simulink model "tb_adc_5g_D3"  (Simulink 7.0)
settings: Solver=ode45  StartTime=0.0  StopTime=2000  RelTol=1e-3
libraries: xbsIndex_r4 x125, simulink x36, dspsigops x20, xps_library x2, casper_library x1
(part 1 of 2)
settings Model: Creator=user  LastModifiedBy=homin
settings DebuggingCC: SaveWithParameterizedLinksMsg=none

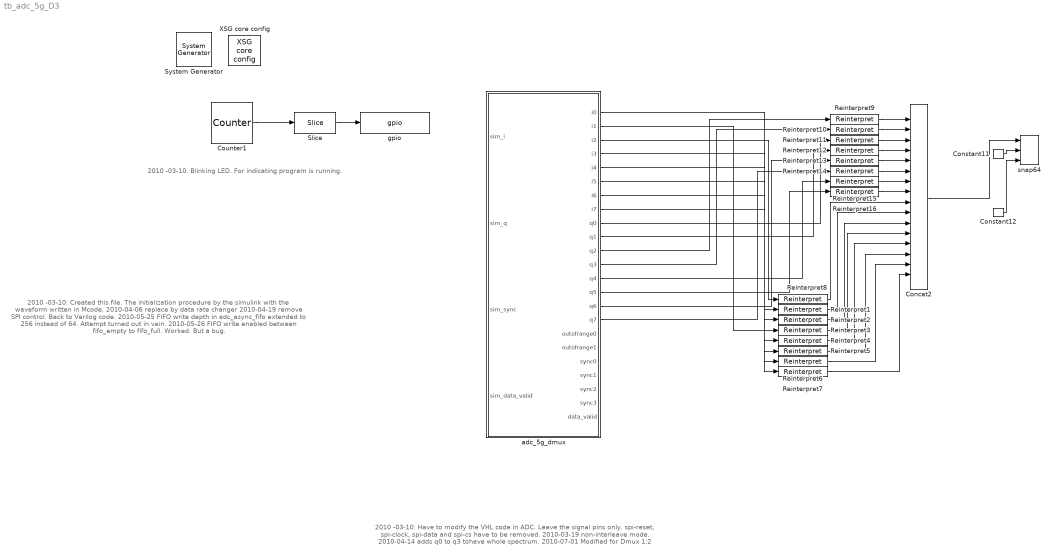
== system tb_adc_5g_D3 ==
  note: 2010 -03-10:
      | Blinking LED. For indicating program is running.
  note: 2010 -03-10:
      | Have to modify the VHL code in ADC. Leave the signal pins only. spi-reset,
      | spi-clock, spi-data and spi-cs have to be removed.
      | 2010-03-19
      | non-interleave mode.
      | 2010-04-14
      | adds q0 to q3 tohave whole spectrum.
      | 2010-07-01
      | Modified for Dmux 1:2
  note: 2010 -03-10:
      | Created this file. The initialization procedure by the simulink with
      | the waveform written in Mcode.
      | 2010-04-06
      | replace by data rate changer
      | 2010-04-19
      | remove SPI control. Back to Verilog code.
      | 2010-05-25
      | FIFO write depth in adc_async_fifo extended to 256 instead of 64. Attempt turned out in vein.
      | 2010-05-26
      | FIFO write enabled between fifo_empty to fifo_full. Worked. But a bug.
  " System Generator" : xbsIndex_r4/ System Generator  Tag=genX  SystemSampleTime=-1  xilinxfamily=virtex5  part=xc5vsx95t  speed=-1  package=ff1136  synthesis_tool=XST  clock_wrapper=Clock Enables  directory=./tb_adc_5g_D3/sysgen  testbench=off  simulink_period=1  sysclk_period=3.3333  dcm_input_clock_period=100  incr_netlist=off  trim_vbits=Everywhere in SubSystem  dbl_ovrd=According to Block Masks  core_generation=According to Block Masks  run_coregen=off  deprecated_control=off  eval_field=0  block_type=sysgen
      settings: block_version=10.1.3
  Concat2 : xbsIndex_r4/Concat  num_inputs=16  dbl_ovrd=off  block_type=concat
      settings: block_version=10.1.3
  Constant11 : xbsIndex_r4/Constant  arith_type=Boolean  const=1  n_bits=16  bin_pt=14  explicit_period=on  period=1  equ=P=C  opselect=C  inp2=PCIN>>17  opr=+  inp1=P  carry=CIN  dbl_ovrd=off  block_type=constant
  Constant12 : xbsIndex_r4/Constant  arith_type=Boolean  const=1  n_bits=16  bin_pt=14  explicit_period=on  period=1  equ=P=C  opselect=C  inp2=PCIN>>17  opr=+  inp1=P  carry=CIN  dbl_ovrd=off  block_type=constant
  Counter1 : xbsIndex_r4/Counter  cnt_type=Free Running  cnt_to=Inf  operation=Up  start_count=0  cnt_by_val=1  arith_type=Unsigned  n_bits=27  bin_pt=0  load_pin=off  rst=off  en=off  explicit_period=on  period=1  dbl_ovrd=off  use_behavioral_HDL=off  use_rpm=off  implementation=Fabric  block_type=counter
  Reinterpret{1..16} (16 alike) : xbsIndex_r4/Reinterpret  force_arith_type=on  arith_type=Unsigned  force_bin_pt=on  bin_pt=0  block_type=reinterpret
      settings: infoedit="Changes signal type without altering the binary representation.   You can changed the signal between signed and unsigned, and relocate the binary point.<P><P>Hardware notes: In hardware this block costs nothing.<P><P>Example:  Suppose the input is 6 bits wide, signed, with 2 fractional bits, and the output is forced to unsigned with 0 fractional bits.  Then an input of -2.0 (1110.00 in binary 2's complement) becomes an output of 56 (111000 in binary)."  block_version=10.1.3
  Slice : xbsIndex_r4/Slice  nbits=1  boolean_output=on  mode=Lower Bit Location + Width  bit1=27  base1=MSB of Input  bit0=26  base0=LSB of Input  dbl_ovrd=off  block_type=slice
      settings: infoedit="Extracts a given range of bits from each input sample and presents it at the output.  The output type is ordinarily unsigned with binary point at zero, but can be Boolean when the slice is one bit wide.<P><P>Hardware notes: In hardware this block costs nothing."  block_version=10.1.3
  XSG core config : xps_library/XSG core config  Tag=xps:xsg  SystemSampleTime=-1  hw_sys=ROACH:sx95t  ibob_linux=off  clk_src=adc0_clk  iBOB_clk_src=sys_clk  BEE2_ctrl_clk_src=sys_clk  BEE2_usr_clk_src=sys_clk  ROACH_clk_src=adc0_clk  CORR_clk_src=sys_clk  gpio_clk_io_group=iBOB:sma  gpio_clk_bit_index=0  clk_rate=300  sample_period=1  synthesis_tool=XST  mpc_type=powerpc440_ext
  adc_5g_dmux : Subsystem  Tag=xps:adc_5g_dmux  mask(adc){adc_brd=adc0, adc_clk_rate=1200, adc_interleave=off, sample_period=1}
      mask prompts: adc_brd "ADC board"; adc_clk_rate "ADC clock rate (MHz)"; adc_interleave "ADC interleave mode"; sample_period "Sample period"
      mask help: The ADC block converts analog inputs to digital outputs. Every clock cycle, the inputs are sampled and digitized to 8 bit binary point numbers in the range of [-1, 1) and are then output by the adc.
      mask init:
      | adc_5g_mask;
      mask Help: eval('xlWeb([getenv(''MLIB_ROOT''), ''\doc\html\sys_adc\sys_adc.html''])')
      mask StyleString: popup(adc0|adc1),edit,checkbox,edit
  gpio : xps_library/gpio  Tag=xps:gpio  SystemSampleTime=-1  io_group=ROACH:led  io_dir=out  arith_type=Boolean  bitwidth=1  bin_pt=0  bit_index=1  sample_period=1  use_single_ended=off  use_ddr=off  reg_iob=on  reg_clk_phase=0  termination=None
      link override convert: arith_type=Boolean  n_bits=1  bin_pt=0
  snap64 : casper_library/Scopes/snap64  SystemSampleTime=-1  nsamples=11
      link override addr/convert: arith_type=Unsigned  n_bits=32  bin_pt=0
      link override bram_lsb/convert_din: arith_type=Unsigned
      link override bram_lsb/mem/sim_data_in: arith_type=Unsigned
      link override bram_lsb/tb_adc_5g_D1_snap64_bram_lsb_data_out: arith_type=Unsigned
      link override bram_lsb/tb_adc_5g_D2_snap64_bram_lsb_data_out: arith_type=Unsigned
      link override bram_lsb/tb_adc_5g_D3_snap64_bram_lsb_data_out: arith_type=Unsigned
      link override bram_lsb/tb_adc_5g_spi_V3_snap64_bram_lsb_data_out: arith_type=Unsigned
      link override bram_lsb/tb_adc_5g_spi_V5_snap64_bram_lsb_data_out: arith_type=Unsigned
      link override bram_lsb/tb_adc_5g_spi_rw2_snap64_bram_lsb_data_out: arith_type=Unsigned
      link override bram_lsb/tut6_snap64_bram_lsb_data_out: arith_type=Unsigned
      link override bram_msb/convert_din: arith_type=Unsigned
      link override bram_msb/mem/sim_data_in: arith_type=Unsigned
      link override bram_msb/tb_adc_5g_D1_snap64_bram_msb_data_out: arith_type=Unsigned
      link override bram_msb/tb_adc_5g_D2_snap64_bram_msb_data_out: arith_type=Unsigned
      link override bram_msb/tb_adc_5g_D3_snap64_bram_msb_data_out: arith_type=Unsigned
      link override bram_msb/tb_adc_5g_spi_V3_snap64_bram_msb_data_out: arith_type=Unsigned
      link override bram_msb/tb_adc_5g_spi_V5_snap64_bram_msb_data_out: arith_type=Unsigned
      link override bram_msb/tb_adc_5g_spi_rw2_snap64_bram_msb_data_out: arith_type=Unsigned
      link override bram_msb/tut6_snap64_bram_msb_data_out: arith_type=Unsigned
      link override ctrl/tb_adc_5g_D1_snap64_ctrl_user_data_out: arith_type=Unsigned  n_bits=32  bin_pt=0  period=1
      link override ctrl/tb_adc_5g_D2_snap64_ctrl_user_data_out: arith_type=Unsigned  n_bits=32  bin_pt=0  period=1
      link override ctrl/tb_adc_5g_D3_snap64_ctrl_user_data_out: arith_type=Unsigned  n_bits=32  bin_pt=0  period=1
      link override ctrl/tb_adc_5g_spi_V3_snap64_ctrl_user_data_out: arith_type=Unsigned  n_bits=32  bin_pt=0  period=1
      link override ctrl/tb_adc_5g_spi_V5_snap64_ctrl_user_data_out: arith_type=Unsigned  n_bits=32  bin_pt=0  period=1
      link override ctrl/tb_adc_5g_spi_rw2_snap64_ctrl_user_data_out: arith_type=Unsigned  n_bits=32  bin_pt=0  period=1
      link override ctrl/tut6_snap64_ctrl_user_data_out: arith_type=Unsigned  n_bits=32  bin_pt=0  period=1
  wires:
  Counter1/1 -> Slice/1
  Slice/1 -> gpio/1
  Reinterpret9/1 -> Concat2/1
  Reinterpret10/1 -> Concat2/2
  Reinterpret11/1 -> Concat2/3
  Reinterpret12/1 -> Concat2/4
  Reinterpret13/1 -> Concat2/5
  Reinterpret14/1 -> Concat2/6
  Reinterpret15/1 -> Concat2/7
  Reinterpret16/1 -> Concat2/8
  Concat2/1 -> snap64/1
  Constant11/1 -> snap64/2
  Constant12/1 -> snap64/3
  Reinterpret8/1 -> Concat2/9
  Reinterpret1/1 -> Concat2/10
  Reinterpret2/1 -> Concat2/11
  Reinterpret3/1 -> Concat2/12
  Reinterpret4/1 -> Concat2/13
  Reinterpret5/1 -> Concat2/14
  Reinterpret6/1 -> Concat2/15
  Reinterpret7/1 -> Concat2/16
  adc_5g_dmux/11(q2) -> Reinterpret9/1
  adc_5g_dmux/12(q3) -> Reinterpret10/1
  adc_5g_dmux/9(q0) -> Reinterpret11/1
  adc_5g_dmux/10(q1) -> Reinterpret12/1
  adc_5g_dmux/13(q4) -> Reinterpret15/1
  adc_5g_dmux/14(q5) -> Reinterpret16/1
  adc_5g_dmux/15(q6) -> Reinterpret13/1
  adc_5g_dmux/16(q7) -> Reinterpret14/1
  adc_5g_dmux/3(i2) -> Reinterpret8/1
  adc_5g_dmux/4(i3) -> Reinterpret1/1
  adc_5g_dmux/1(i0) -> Reinterpret2/1
  adc_5g_dmux/2(i1) -> Reinterpret3/1
  adc_5g_dmux/7(i6) -> Reinterpret4/1
  adc_5g_dmux/8(i7) -> Reinterpret5/1
  adc_5g_dmux/5(i4) -> Reinterpret6/1
  adc_5g_dmux/6(i5) -> Reinterpret7/1

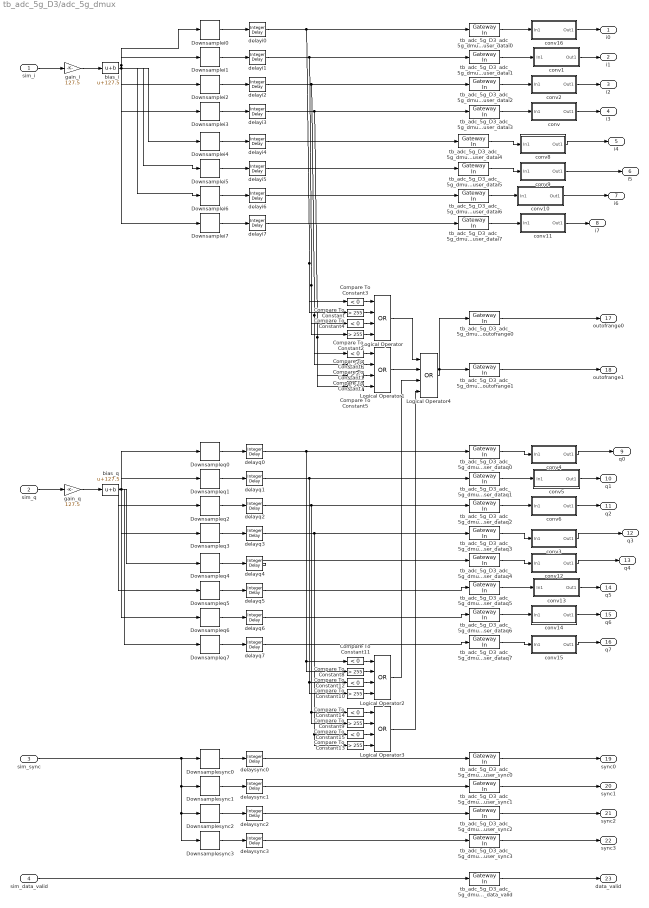
== system tb_adc_5g_D3/adc_5g_dmux ==
  sim_i : Inport  SampleTime=sample_period/4
  sim_q : Inport  Port=2  SampleTime=sample_period/4
  sim_sync : Inport  Port=3  SampleTime=sample_period/4  OutDataType=sfix(16)  OutScaling=2^0
  sim_data_valid : Inport  Port=4  SampleTime=sample_period/4  OutDataType=sfix(16)  OutScaling=2^0
  Compare To Constant{,1..2,5,8..10,13} (8 alike) : simulink/Logic and Bit Operations/Compare To Constant  SystemSampleTime=-1  relop=>  const=255  LogicOutDataTypeMode=boolean  ZeroCross=off
  Compare To Constant{3..4,6..7,11..12,14..15} (8 alike) : simulink/Logic and Bit Operations/Compare To Constant  SystemSampleTime=-1  relop=<  const=0  LogicOutDataTypeMode=boolean  ZeroCross=off
  Downsamplei0 : dspsigops/Downsample  N=4  phase=0  ic=0  smode=Allow multirate  fmode=Maintain input frame size
  Downsamplei1 : dspsigops/Downsample  N=4  phase=1  ic=0  smode=Allow multirate  fmode=Maintain input frame size
  Downsamplei2 : dspsigops/Downsample  N=4  phase=2  ic=0  smode=Allow multirate  fmode=Maintain input frame size
  Downsamplei3 : dspsigops/Downsample  N=4  phase=3  ic=0  smode=Allow multirate  fmode=Maintain input frame size
  Downsamplei4 : dspsigops/Downsample  N=4  phase=0  ic=0  smode=Allow multirate  fmode=Maintain input frame size
  Downsamplei5 : dspsigops/Downsample  N=4  phase=1  ic=0  smode=Allow multirate  fmode=Maintain input frame size
  Downsamplei6 : dspsigops/Downsample  N=4  phase=2  ic=0  smode=Allow multirate  fmode=Maintain input frame size
  Downsamplei7 : dspsigops/Downsample  N=4  phase=3  ic=0  smode=Allow multirate  fmode=Maintain input frame size
  Downsampleq0 : dspsigops/Downsample  N=4  phase=0  ic=0  smode=Allow multirate  fmode=Maintain input frame size
  Downsampleq1 : dspsigops/Downsample  N=4  phase=1  ic=0  smode=Allow multirate  fmode=Maintain input frame size
  Downsampleq2 : dspsigops/Downsample  N=4  phase=2  ic=0  smode=Allow multirate  fmode=Maintain input frame size
  Downsampleq3 : dspsigops/Downsample  N=4  phase=3  ic=0  smode=Allow multirate  fmode=Maintain input frame size
  Downsampleq4 : dspsigops/Downsample  N=4  phase=0  ic=0  smode=Allow multirate  fmode=Maintain input frame size
  Downsampleq5 : dspsigops/Downsample  N=4  phase=1  ic=0  smode=Allow multirate  fmode=Maintain input frame size
  Downsampleq6 : dspsigops/Downsample  N=4  phase=2  ic=0  smode=Allow multirate  fmode=Maintain input frame size
  Downsampleq7 : dspsigops/Downsample  N=4  phase=3  ic=0  smode=Allow multirate  fmode=Maintain input frame size
  Downsamplesync0 : dspsigops/Downsample  N=4  phase=0  ic=0  smode=Allow multirate  fmode=Maintain input frame size
  Downsamplesync1 : dspsigops/Downsample  N=4  phase=1  ic=0  smode=Allow multirate  fmode=Maintain input frame size
  Downsamplesync2 : dspsigops/Downsample  N=4  phase=2  ic=0  smode=Allow multirate  fmode=Maintain input frame size
  Downsamplesync3 : dspsigops/Downsample  N=4  phase=3  ic=0  smode=Allow multirate  fmode=Maintain input frame size
  Logical Operator{,1..4} (5 alike) : Logic  Operator=OR  Inputs=4  AllPortsSameDT=off  OutDataTypeMode=boolean
  bias_i : Bias  Bias=127.5  SaturateOnIntegerOverflow=on
  bias_q : Bias  Bias=127.5  SaturateOnIntegerOverflow=on
  conv : Subsystem
  conv1 : Subsystem
  conv10 : Subsystem
  conv11 : Subsystem
  conv12 : Subsystem
  conv13 : Subsystem
  conv14 : Subsystem
  conv15 : Subsystem
  conv16 : Subsystem
  conv2 : Subsystem
  conv3 : Subsystem
  conv4 : Subsystem
  conv5 : Subsystem
  conv6 : Subsystem
  conv8 : Subsystem
  conv9 : Subsystem
  delayi0 : simulink/Discrete/Integer Delay  vinit=0.0  samptime=-1  NumDelays=2
  delayi{1..3,5..7} (6 alike) : simulink/Discrete/Integer Delay  vinit=0.0  samptime=-1  NumDelays=1
  delayi4 : simulink/Discrete/Integer Delay  vinit=0.0  samptime=-1  NumDelays=2
  delayq0 : simulink/Discrete/Integer Delay  vinit=0.0  samptime=-1  NumDelays=2
  delayq{1..3,5..7} (6 alike) : simulink/Discrete/Integer Delay  vinit=0.0  samptime=-1  NumDelays=1
  delayq4 : simulink/Discrete/Integer Delay  vinit=0.0  samptime=-1  NumDelays=2
  delaysync0 : simulink/Discrete/Integer Delay  vinit=0.0  samptime=-1  NumDelays=2
  delaysync1 : simulink/Discrete/Integer Delay  vinit=0.0  samptime=-1  NumDelays=1
  delaysync2 : simulink/Discrete/Integer Delay  vinit=0.0  samptime=-1  NumDelays=1
  delaysync3 : simulink/Discrete/Integer Delay  vinit=0.0  samptime=-1  NumDelays=1
  gain_i : Gain  Gain=127.5  SaturateOnIntegerOverflow=on
  gain_q : Gain  Gain=127.5  SaturateOnIntegerOverflow=on
  tb_adc_5g_D3_adc_5g_dmux_user_data_valid : xbsIndex_r4/Gateway In  arith_type=Boolean  n_bits=8  bin_pt=0  quantization="Round  (unbiased: +/- Inf)"  overflow=Saturate  period=sample_period  dbl_ovrd=off  timing_constraint=None  locs_specified=off  LOCs={}  block_type=gatewayin
      settings: infoedit="Gateway in block.  Converts inputs of type Simulink integer, double and fixed point to  Xilinx fixed point type.<P><P>Hardware notes:  In hardware these blocks become top level input ports."  xl_area=[0 0 0 0 8 0 0]  block_version=8.2.02
  tb_adc_5g_D3_adc_5g_dmux_user_datai{0..7} (8 alike) : xbsIndex_r4/Gateway In  arith_type=Unsigned  n_bits=4  bin_pt=0  quantization="Round  (unbiased: +/- Inf)"  overflow=Saturate  period=sample_period  dbl_ovrd=off  timing_constraint=None  locs_specified=off  LOCs={}  block_type=gatewayin
      settings: infoedit="Gateway in block.  Converts inputs of type Simulink integer, double and fixed point to  Xilinx fixed point type.<P><P>Hardware notes:  In hardware these blocks become top level input ports."  xl_area=[0 0 0 0 8 0 0]  block_version=8.2.02
  tb_adc_5g_D3_adc_5g_dmux_user_dataq{0..7} (8 alike) : xbsIndex_r4/Gateway In  arith_type=Unsigned  n_bits=4  bin_pt=0  quantization="Round  (unbiased: +/- Inf)"  overflow=Saturate  period=sample_period  dbl_ovrd=off  timing_constraint=None  locs_specified=off  LOCs={}  block_type=gatewayin
      settings: infoedit="Gateway in block.  Converts inputs of type Simulink integer, double and fixed point to  Xilinx fixed point type.<P><P>Hardware notes:  In hardware these blocks become top level input ports."  xl_area=[0 0 0 0 8 0 0]  block_version=8.2.02
  tb_adc_5g_D3_adc_5g_dmux_user_outofrange0 : xbsIndex_r4/Gateway In  arith_type=Boolean  n_bits=8  bin_pt=0  quantization="Round  (unbiased: +/- Inf)"  overflow=Saturate  period=sample_period  dbl_ovrd=off  timing_constraint=None  locs_specified=off  LOCs={}  block_type=gatewayin
      settings: infoedit="Gateway in block.  Converts inputs of type Simulink integer, double and fixed point to  Xilinx fixed point type.<P><P>Hardware notes:  In hardware these blocks become top level input ports."  xl_area=[0 0 0 0 8 0 0]  block_version=8.2.02
  tb_adc_5g_D3_adc_5g_dmux_user_outofrange1 : xbsIndex_r4/Gateway In  arith_type=Boolean  n_bits=8  bin_pt=0  quantization="Round  (unbiased: +/- Inf)"  overflow=Saturate  period=sample_period  dbl_ovrd=off  timing_constraint=None  locs_specified=off  LOCs={}  block_type=gatewayin
      settings: infoedit="Gateway in block.  Converts inputs of type Simulink integer, double and fixed point to  Xilinx fixed point type.<P><P>Hardware notes:  In hardware these blocks become top level input ports."  xl_area=[0 0 0 0 8 0 0]  block_version=8.2.02
  tb_adc_5g_D3_adc_5g_dmux_user_sync{0..3} (4 alike) : xbsIndex_r4/Gateway In  arith_type=Boolean  n_bits=8  bin_pt=0  quantization="Round  (unbiased: +/- Inf)"  overflow=Saturate  period=sample_period  dbl_ovrd=off  timing_constraint=None  locs_specified=off  LOCs={}  block_type=gatewayin
      settings: infoedit="Gateway in block.  Converts inputs of type Simulink integer, double and fixed point to  Xilinx fixed point type.<P><P>Hardware notes:  In hardware these blocks become top level input ports."  xl_area=[0 0 0 0 8 0 0]  block_version=8.2.02
  i0 : Outport  OutDataType=sfix(16)  OutScaling=2^0
  i1 : Outport  Port=2  OutDataType=sfix(16)  OutScaling=2^0
  i2 : Outport  Port=3  OutDataType=sfix(16)  OutScaling=2^0
  i3 : Outport  Port=4  OutDataType=sfix(16)  OutScaling=2^0
  i4 : Outport  Port=5  OutDataType=sfix(16)  OutScaling=2^0
  i5 : Outport  Port=6  OutDataType=sfix(16)  OutScaling=2^0
  i6 : Outport  Port=7  OutDataType=sfix(16)  OutScaling=2^0
  i7 : Outport  Port=8  OutDataType=sfix(16)  OutScaling=2^0
  q0 : Outport  Port=9  OutDataType=sfix(16)  OutScaling=2^0
  q1 : Outport  Port=10  OutDataType=sfix(16)  OutScaling=2^0
  q2 : Outport  Port=11  OutDataType=sfix(16)  OutScaling=2^0
  q3 : Outport  Port=12  OutDataType=sfix(16)  OutScaling=2^0
  q4 : Outport  Port=13  OutDataType=sfix(16)  OutScaling=2^0
  q5 : Outport  Port=14  OutDataType=sfix(16)  OutScaling=2^0
  q6 : Outport  Port=15  OutDataType=sfix(16)  OutScaling=2^0
  q7 : Outport  Port=16  OutDataType=sfix(16)  OutScaling=2^0
  outofrange0 : Outport  Port=17  OutDataType=sfix(16)  OutScaling=2^0
  outofrange1 : Outport  Port=18  OutDataType=sfix(16)  OutScaling=2^0
  sync0 : Outport  Port=19  OutDataType=sfix(16)  OutScaling=2^0
  sync1 : Outport  Port=20  OutDataType=sfix(16)  OutScaling=2^0
  sync2 : Outport  Port=21  OutDataType=sfix(16)  OutScaling=2^0
  sync3 : Outport  Port=22  OutDataType=sfix(16)  OutScaling=2^0
  data_valid : Outport  Port=23  OutDataType=sfix(16)  OutScaling=2^0
  wires:
  tb_adc_5g_D3_adc_5g_dmux_user_datai0/1 -> conv16/1(In1)
  sim_data_valid/1 -> tb_adc_5g_D3_adc_5g_dmux_user_data_valid/1
  tb_adc_5g_D3_adc_5g_dmux_user_data_valid/1 -> data_valid/1
  tb_adc_5g_D3_adc_5g_dmux_user_sync3/1 -> sync3/1
  tb_adc_5g_D3_adc_5g_dmux_user_sync2/1 -> sync2/1
  delaysync3/1 -> tb_adc_5g_D3_adc_5g_dmux_user_sync3/1
  delaysync2/1 -> tb_adc_5g_D3_adc_5g_dmux_user_sync2/1
  Downsamplesync3/1 -> delaysync3/1
  Downsamplesync2/1 -> delaysync2/1
  tb_adc_5g_D3_adc_5g_dmux_user_sync1/1 -> sync1/1
  delaysync0/1 -> tb_adc_5g_D3_adc_5g_dmux_user_sync0/1
  Downsamplesync1/1 -> delaysync1/1
  Downsamplesync0/1 -> delaysync0/1
  sim_sync/1 -> Downsamplesync3/1, Downsamplesync2/1, Downsamplesync1/1, Downsamplesync0/1
  Compare To Constant5/1 -> Logical Operator1/4
  Compare To Constant7/1 -> Logical Operator1/3
  Compare To Constant1/1 -> Logical Operator1/2
  Compare To Constant6/1 -> Logical Operator1/1
  Compare To Constant2/1 -> Logical Operator/4
  Compare To Constant4/1 -> Logical Operator/3
  Compare To Constant/1 -> Logical Operator/2
  Compare To Constant3/1 -> Logical Operator/1
  tb_adc_5g_D3_adc_5g_dmux_user_outofrange1/1 -> outofrange1/1
  delayq0/1 -> tb_adc_5g_D3_adc_5g_dmux_user_dataq0/1, Compare To Constant8/1, Compare To Constant11/1
  Downsampleq0/1 -> delayq0/1
  delayi0/1 -> Compare To Constant3/1, Compare To Constant/1, tb_adc_5g_D3_adc_5g_dmux_user_datai0/1
  Downsamplei1/1 -> delayi1/1
  Downsamplei2/1 -> delayi2/1
  Downsamplei3/1 -> delayi3/1
  Downsampleq1/1 -> delayq1/1
  Downsampleq2/1 -> delayq2/1
  Downsampleq3/1 -> delayq3/1
  tb_adc_5g_D3_adc_5g_dmux_user_datai1/1 -> conv1/1(In1)
  tb_adc_5g_D3_adc_5g_dmux_user_datai2/1 -> conv2/1(In1)
  tb_adc_5g_D3_adc_5g_dmux_user_datai3/1 -> conv/1(In1)
  tb_adc_5g_D3_adc_5g_dmux_user_outofrange0/1 -> outofrange0/1
  tb_adc_5g_D3_adc_5g_dmux_user_sync0/1 -> sync0/1
  conv16/1(Out1) -> i0/1
  conv1/1(Out1) -> i1/1
  conv2/1(Out1) -> i2/1
  conv/1(Out1) -> i3/1
  tb_adc_5g_D3_adc_5g_dmux_user_dataq0/1 -> conv4/1(In1)
  conv4/1(Out1) -> q0/1
  tb_adc_5g_D3_adc_5g_dmux_user_dataq1/1 -> conv5/1(In1)
  conv5/1(Out1) -> q1/1
  tb_adc_5g_D3_adc_5g_dmux_user_dataq2/1 -> conv6/1(In1)
  conv6/1(Out1) -> q2/1
  tb_adc_5g_D3_adc_5g_dmux_user_dataq3/1 -> conv3/1(In1)
  conv3/1(Out1) -> q3/1
  Downsamplei0/1 -> delayi0/1
  delayi1/1 -> Compare To Constant4/1, Compare To Constant2/1, tb_adc_5g_D3_adc_5g_dmux_user_datai1/1
  delayi2/1 -> Compare To Constant1/1, Compare To Constant6/1, tb_adc_5g_D3_adc_5g_dmux_user_datai2/1
  delayi3/1 -> Compare To Constant5/1, Compare To Constant7/1, tb_adc_5g_D3_adc_5g_dmux_user_datai3/1
  delayq1/1 -> Compare To Constant10/1, Compare To Constant12/1, tb_adc_5g_D3_adc_5g_dmux_user_dataq1/1
  delayq2/1 -> Compare To Constant9/1, Compare To Constant14/1, tb_adc_5g_D3_adc_5g_dmux_user_dataq2/1
  delayq3/1 -> Compare To Constant13/1, Compare To Constant15/1, tb_adc_5g_D3_adc_5g_dmux_user_dataq3/1
  delaysync1/1 -> tb_adc_5g_D3_adc_5g_dmux_user_sync1/1
  Compare To Constant11/1 -> Logical Operator2/1
  Compare To Constant13/1 -> Logical Operator3/4
  Compare To Constant15/1 -> Logical Operator3/3
  Compare To Constant9/1 -> Logical Operator3/2
  Compare To Constant14/1 -> Logical Operator3/1
  Compare To Constant10/1 -> Logical Operator2/4
  Compare To Constant12/1 -> Logical Operator2/3
  Compare To Constant8/1 -> Logical Operator2/2
  Logical Operator4/1 -> tb_adc_5g_D3_adc_5g_dmux_user_outofrange0/1, tb_adc_5g_D3_adc_5g_dmux_user_outofrange1/1
  Logical Operator/1 -> Logical Operator4/1
  Logical Operator1/1 -> Logical Operator4/2
  Logical Operator2/1 -> Logical Operator4/3
  Logical Operator3/1 -> Logical Operator4/4
  sim_i/1 -> gain_i/1
  gain_i/1 -> bias_i/1
  bias_i/1 -> Downsamplei1/1, Downsamplei2/1, Downsamplei3/1, Downsamplei4/1, Downsamplei5/1, Downsamplei6/1, Downsamplei0/1, Downsamplei7/1
  sim_q/1 -> gain_q/1
  gain_q/1 -> bias_q/1
  bias_q/1 -> Downsampleq0/1, Downsampleq1/1, Downsampleq3/1, Downsampleq4/1, Downsampleq2/1, Downsampleq5/1, Downsampleq6/1, Downsampleq7/1
  tb_adc_5g_D3_adc_5g_dmux_user_datai4/1 -> conv8/1(In1)
  delayi4/1 -> tb_adc_5g_D3_adc_5g_dmux_user_datai4/1
  tb_adc_5g_D3_adc_5g_dmux_user_datai5/1 -> conv9/1(In1)
  tb_adc_5g_D3_adc_5g_dmux_user_datai6/1 -> conv10/1(In1)
  tb_adc_5g_D3_adc_5g_dmux_user_datai7/1 -> conv11/1(In1)
  conv8/1(Out1) -> i4/1
  conv9/1(Out1) -> i5/1
  conv10/1(Out1) -> i6/1
  conv11/1(Out1) -> i7/1
  delayi5/1 -> tb_adc_5g_D3_adc_5g_dmux_user_datai5/1
  delayi6/1 -> tb_adc_5g_D3_adc_5g_dmux_user_datai6/1
  delayi7/1 -> tb_adc_5g_D3_adc_5g_dmux_user_datai7/1
  Downsamplei5/1 -> delayi5/1
  Downsamplei6/1 -> delayi6/1
  Downsamplei7/1 -> delayi7/1
  Downsamplei4/1 -> delayi4/1
  tb_adc_5g_D3_adc_5g_dmux_user_dataq4/1 -> conv12/1(In1)
  conv12/1(Out1) -> q4/1
  tb_adc_5g_D3_adc_5g_dmux_user_dataq5/1 -> conv13/1(In1)
  conv13/1(Out1) -> q5/1
  tb_adc_5g_D3_adc_5g_dmux_user_dataq6/1 -> conv14/1(In1)
  conv14/1(Out1) -> q6/1
  tb_adc_5g_D3_adc_5g_dmux_user_dataq7/1 -> conv15/1(In1)
  conv15/1(Out1) -> q7/1
  Downsampleq4/1 -> delayq4/1
  Downsampleq5/1 -> delayq5/1
  Downsampleq6/1 -> delayq6/1
  Downsampleq7/1 -> delayq7/1
  delayq4/1 -> tb_adc_5g_D3_adc_5g_dmux_user_dataq4/1
  delayq5/1 -> tb_adc_5g_D3_adc_5g_dmux_user_dataq5/1
  delayq6/1 -> tb_adc_5g_D3_adc_5g_dmux_user_dataq6/1
  delayq7/1 -> tb_adc_5g_D3_adc_5g_dmux_user_dataq7/1

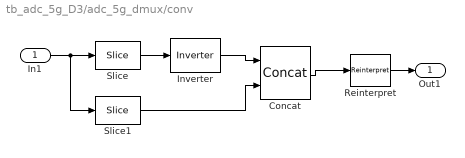
== system tb_adc_5g_D3/adc_5g_dmux/conv ==
  In1 : Inport  OutDataType=sfix(16)  OutScaling=2^0
  Concat : xbsIndex_r4/Concat  num_inputs=2  dbl_ovrd=off  block_type=concat
      settings: block_version=8.2.02
  Inverter : xbsIndex_r4/Inverter  en=off  latency=0  dbl_ovrd=off  block_type=inv
      settings: xl_area=[0, 0, 0, 0, 0, 0, 0]  block_version=8.2.02
  Reinterpret : xbsIndex_r4/Reinterpret  force_arith_type=on  arith_type="Signed  (2's comp)"  force_bin_pt=on  bin_pt=3  block_type=reinterpret
      settings: infoedit="Changes signal type without altering the binary representation.   You can changed the signal between signed and unsigned, and relocate the binary point.<P><P>Hardware notes: In hardware this block costs nothing.<P><P>Example:  Suppose the input is 6 bits wide, signed, with 2 fractional bits, and the output is forced to unsigned with 0 fractional bits.  Then an input of -2.0 (1110.00 in binary 2's complement) becomes an output of 56 (111000 in binary)."  block_version=8.2.02
  Slice : xbsIndex_r4/Slice  nbits=1  boolean_output=off  mode=Upper Bit Location + Width  bit1=0  base1=MSB of Input  bit0=0  base0=LSB of Input  dbl_ovrd=off  block_type=slice
      settings: infoedit="Extracts a given range of bits from each input sample and presents it at the output.  The output type is ordinarily unsigned with binary point at zero, but can be Boolean when the slice is one bit wide.<P><P>Hardware notes: In hardware this block costs nothing."  block_version=8.2.02
  Slice1 : xbsIndex_r4/Slice  nbits=3  boolean_output=off  mode=Lower Bit Location + Width  bit1=0  base1=MSB of Input  bit0=0  base0=LSB of Input  dbl_ovrd=off  block_type=slice
      settings: infoedit="Extracts a given range of bits from each input sample and presents it at the output.  The output type is ordinarily unsigned with binary point at zero, but can be Boolean when the slice is one bit wide.<P><P>Hardware notes: In hardware this block costs nothing."  block_version=8.2.02
  Out1 : Outport  OutDataType=sfix(16)  OutScaling=2^0
  wires:
  In1/1 -> Slice1/1, Slice/1
  Slice/1 -> Inverter/1
  Inverter/1 -> Concat/1
  Slice1/1 -> Concat/2
  Concat/1 -> Reinterpret/1
  Reinterpret/1 -> Out1/1

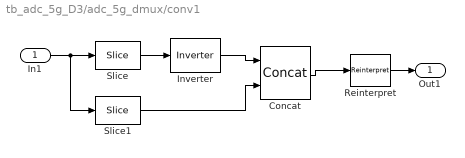
== system tb_adc_5g_D3/adc_5g_dmux/conv1 ==
  In1 : Inport  OutDataType=sfix(16)  OutScaling=2^0
  Concat : xbsIndex_r4/Concat  num_inputs=2  dbl_ovrd=off  block_type=concat
      settings: block_version=8.2.02
  Inverter : xbsIndex_r4/Inverter  en=off  latency=0  dbl_ovrd=off  block_type=inv
      settings: xl_area=[0, 0, 0, 0, 0, 0, 0]  block_version=8.2.02
  Reinterpret : xbsIndex_r4/Reinterpret  force_arith_type=on  arith_type="Signed  (2's comp)"  force_bin_pt=on  bin_pt=3  block_type=reinterpret
      settings: infoedit="Changes signal type without altering the binary representation.   You can changed the signal between signed and unsigned, and relocate the binary point.<P><P>Hardware notes: In hardware this block costs nothing.<P><P>Example:  Suppose the input is 6 bits wide, signed, with 2 fractional bits, and the output is forced to unsigned with 0 fractional bits.  Then an input of -2.0 (1110.00 in binary 2's complement) becomes an output of 56 (111000 in binary)."  block_version=8.2.02
  Slice : xbsIndex_r4/Slice  nbits=1  boolean_output=off  mode=Upper Bit Location + Width  bit1=0  base1=MSB of Input  bit0=0  base0=LSB of Input  dbl_ovrd=off  block_type=slice
      settings: infoedit="Extracts a given range of bits from each input sample and presents it at the output.  The output type is ordinarily unsigned with binary point at zero, but can be Boolean when the slice is one bit wide.<P><P>Hardware notes: In hardware this block costs nothing."  block_version=8.2.02
  Slice1 : xbsIndex_r4/Slice  nbits=3  boolean_output=off  mode=Lower Bit Location + Width  bit1=0  base1=MSB of Input  bit0=0  base0=LSB of Input  dbl_ovrd=off  block_type=slice
      settings: infoedit="Extracts a given range of bits from each input sample and presents it at the output.  The output type is ordinarily unsigned with binary point at zero, but can be Boolean when the slice is one bit wide.<P><P>Hardware notes: In hardware this block costs nothing."  block_version=8.2.02
  Out1 : Outport  OutDataType=sfix(16)  OutScaling=2^0
  wires:
  In1/1 -> Slice1/1, Slice/1
  Slice/1 -> Inverter/1
  Inverter/1 -> Concat/1
  Slice1/1 -> Concat/2
  Concat/1 -> Reinterpret/1
  Reinterpret/1 -> Out1/1

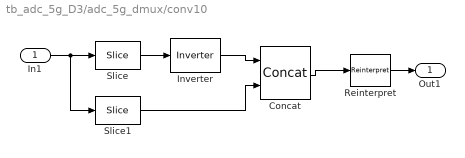
== system tb_adc_5g_D3/adc_5g_dmux/conv10 ==
  In1 : Inport  OutDataType=sfix(16)  OutScaling=2^0
  Concat : xbsIndex_r4/Concat  num_inputs=2  dbl_ovrd=off  block_type=concat
      settings: block_version=8.2.02
  Inverter : xbsIndex_r4/Inverter  en=off  latency=0  dbl_ovrd=off  block_type=inv
      settings: xl_area=[0, 0, 0, 0, 0, 0, 0]  block_version=8.2.02
  Reinterpret : xbsIndex_r4/Reinterpret  force_arith_type=on  arith_type="Signed  (2's comp)"  force_bin_pt=on  bin_pt=3  block_type=reinterpret
      settings: infoedit="Changes signal type without altering the binary representation.   You can changed the signal between signed and unsigned, and relocate the binary point.<P><P>Hardware notes: In hardware this block costs nothing.<P><P>Example:  Suppose the input is 6 bits wide, signed, with 2 fractional bits, and the output is forced to unsigned with 0 fractional bits.  Then an input of -2.0 (1110.00 in binary 2's complement) becomes an output of 56 (111000 in binary)."  block_version=8.2.02
  Slice : xbsIndex_r4/Slice  nbits=1  boolean_output=off  mode=Upper Bit Location + Width  bit1=0  base1=MSB of Input  bit0=0  base0=LSB of Input  dbl_ovrd=off  block_type=slice
      settings: infoedit="Extracts a given range of bits from each input sample and presents it at the output.  The output type is ordinarily unsigned with binary point at zero, but can be Boolean when the slice is one bit wide.<P><P>Hardware notes: In hardware this block costs nothing."  block_version=8.2.02
  Slice1 : xbsIndex_r4/Slice  nbits=3  boolean_output=off  mode=Lower Bit Location + Width  bit1=0  base1=MSB of Input  bit0=0  base0=LSB of Input  dbl_ovrd=off  block_type=slice
      settings: infoedit="Extracts a given range of bits from each input sample and presents it at the output.  The output type is ordinarily unsigned with binary point at zero, but can be Boolean when the slice is one bit wide.<P><P>Hardware notes: In hardware this block costs nothing."  block_version=8.2.02
  Out1 : Outport  OutDataType=sfix(16)  OutScaling=2^0
  wires:
  In1/1 -> Slice1/1, Slice/1
  Slice/1 -> Inverter/1
  Inverter/1 -> Concat/1
  Slice1/1 -> Concat/2
  Concat/1 -> Reinterpret/1
  Reinterpret/1 -> Out1/1

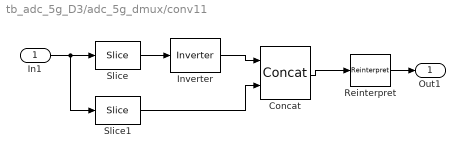
== system tb_adc_5g_D3/adc_5g_dmux/conv11 ==
  In1 : Inport  OutDataType=sfix(16)  OutScaling=2^0
  Concat : xbsIndex_r4/Concat  num_inputs=2  dbl_ovrd=off  block_type=concat
      settings: block_version=8.2.02
  Inverter : xbsIndex_r4/Inverter  en=off  latency=0  dbl_ovrd=off  block_type=inv
      settings: xl_area=[0, 0, 0, 0, 0, 0, 0]  block_version=8.2.02
  Reinterpret : xbsIndex_r4/Reinterpret  force_arith_type=on  arith_type="Signed  (2's comp)"  force_bin_pt=on  bin_pt=3  block_type=reinterpret
      settings: infoedit="Changes signal type without altering the binary representation.   You can changed the signal between signed and unsigned, and relocate the binary point.<P><P>Hardware notes: In hardware this block costs nothing.<P><P>Example:  Suppose the input is 6 bits wide, signed, with 2 fractional bits, and the output is forced to unsigned with 0 fractional bits.  Then an input of -2.0 (1110.00 in binary 2's complement) becomes an output of 56 (111000 in binary)."  block_version=8.2.02
  Slice : xbsIndex_r4/Slice  nbits=1  boolean_output=off  mode=Upper Bit Location + Width  bit1=0  base1=MSB of Input  bit0=0  base0=LSB of Input  dbl_ovrd=off  block_type=slice
      settings: infoedit="Extracts a given range of bits from each input sample and presents it at the output.  The output type is ordinarily unsigned with binary point at zero, but can be Boolean when the slice is one bit wide.<P><P>Hardware notes: In hardware this block costs nothing."  block_version=8.2.02
  Slice1 : xbsIndex_r4/Slice  nbits=3  boolean_output=off  mode=Lower Bit Location + Width  bit1=0  base1=MSB of Input  bit0=0  base0=LSB of Input  dbl_ovrd=off  block_type=slice
      settings: infoedit="Extracts a given range of bits from each input sample and presents it at the output.  The output type is ordinarily unsigned with binary point at zero, but can be Boolean when the slice is one bit wide.<P><P>Hardware notes: In hardware this block costs nothing."  block_version=8.2.02
  Out1 : Outport  OutDataType=sfix(16)  OutScaling=2^0
  wires:
  In1/1 -> Slice1/1, Slice/1
  Slice/1 -> Inverter/1
  Inverter/1 -> Concat/1
  Slice1/1 -> Concat/2
  Concat/1 -> Reinterpret/1
  Reinterpret/1 -> Out1/1

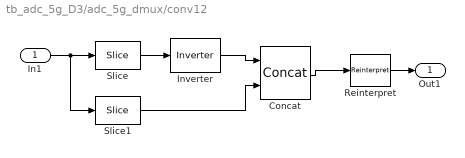
== system tb_adc_5g_D3/adc_5g_dmux/conv12 ==
  In1 : Inport  OutDataType=sfix(16)  OutScaling=2^0
  Concat : xbsIndex_r4/Concat  num_inputs=2  dbl_ovrd=off  block_type=concat
      settings: block_version=8.2.02
  Inverter : xbsIndex_r4/Inverter  en=off  latency=0  dbl_ovrd=off  block_type=inv
      settings: xl_area=[0, 0, 0, 0, 0, 0, 0]  block_version=8.2.02
  Reinterpret : xbsIndex_r4/Reinterpret  force_arith_type=on  arith_type="Signed  (2's comp)"  force_bin_pt=on  bin_pt=3  block_type=reinterpret
      settings: infoedit="Changes signal type without altering the binary representation.   You can changed the signal between signed and unsigned, and relocate the binary point.<P><P>Hardware notes: In hardware this block costs nothing.<P><P>Example:  Suppose the input is 6 bits wide, signed, with 2 fractional bits, and the output is forced to unsigned with 0 fractional bits.  Then an input of -2.0 (1110.00 in binary 2's complement) becomes an output of 56 (111000 in binary)."  block_version=8.2.02
  Slice : xbsIndex_r4/Slice  nbits=1  boolean_output=off  mode=Upper Bit Location + Width  bit1=0  base1=MSB of Input  bit0=0  base0=LSB of Input  dbl_ovrd=off  block_type=slice
      settings: infoedit="Extracts a given range of bits from each input sample and presents it at the output.  The output type is ordinarily unsigned with binary point at zero, but can be Boolean when the slice is one bit wide.<P><P>Hardware notes: In hardware this block costs nothing."  block_version=8.2.02
  Slice1 : xbsIndex_r4/Slice  nbits=3  boolean_output=off  mode=Lower Bit Location + Width  bit1=0  base1=MSB of Input  bit0=0  base0=LSB of Input  dbl_ovrd=off  block_type=slice
      settings: infoedit="Extracts a given range of bits from each input sample and presents it at the output.  The output type is ordinarily unsigned with binary point at zero, but can be Boolean when the slice is one bit wide.<P><P>Hardware notes: In hardware this block costs nothing."  block_version=8.2.02
  Out1 : Outport  OutDataType=sfix(16)  OutScaling=2^0
  wires:
  In1/1 -> Slice1/1, Slice/1
  Slice/1 -> Inverter/1
  Inverter/1 -> Concat/1
  Slice1/1 -> Concat/2
  Concat/1 -> Reinterpret/1
  Reinterpret/1 -> Out1/1

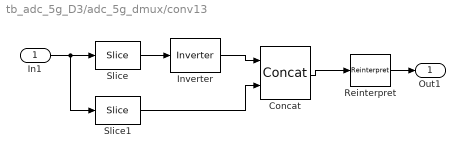
== system tb_adc_5g_D3/adc_5g_dmux/conv13 ==
  In1 : Inport  OutDataType=sfix(16)  OutScaling=2^0
  Concat : xbsIndex_r4/Concat  num_inputs=2  dbl_ovrd=off  block_type=concat
      settings: block_version=8.2.02
  Inverter : xbsIndex_r4/Inverter  en=off  latency=0  dbl_ovrd=off  block_type=inv
      settings: xl_area=[0, 0, 0, 0, 0, 0, 0]  block_version=8.2.02
  Reinterpret : xbsIndex_r4/Reinterpret  force_arith_type=on  arith_type="Signed  (2's comp)"  force_bin_pt=on  bin_pt=3  block_type=reinterpret
      settings: infoedit="Changes signal type without altering the binary representation.   You can changed the signal between signed and unsigned, and relocate the binary point.<P><P>Hardware notes: In hardware this block costs nothing.<P><P>Example:  Suppose the input is 6 bits wide, signed, with 2 fractional bits, and the output is forced to unsigned with 0 fractional bits.  Then an input of -2.0 (1110.00 in binary 2's complement) becomes an output of 56 (111000 in binary)."  block_version=8.2.02
  Slice : xbsIndex_r4/Slice  nbits=1  boolean_output=off  mode=Upper Bit Location + Width  bit1=0  base1=MSB of Input  bit0=0  base0=LSB of Input  dbl_ovrd=off  block_type=slice
      settings: infoedit="Extracts a given range of bits from each input sample and presents it at the output.  The output type is ordinarily unsigned with binary point at zero, but can be Boolean when the slice is one bit wide.<P><P>Hardware notes: In hardware this block costs nothing."  block_version=8.2.02
  Slice1 : xbsIndex_r4/Slice  nbits=3  boolean_output=off  mode=Lower Bit Location + Width  bit1=0  base1=MSB of Input  bit0=0  base0=LSB of Input  dbl_ovrd=off  block_type=slice
      settings: infoedit="Extracts a given range of bits from each input sample and presents it at the output.  The output type is ordinarily unsigned with binary point at zero, but can be Boolean when the slice is one bit wide.<P><P>Hardware notes: In hardware this block costs nothing."  block_version=8.2.02
  Out1 : Outport  OutDataType=sfix(16)  OutScaling=2^0
  wires:
  In1/1 -> Slice1/1, Slice/1
  Slice/1 -> Inverter/1
  Inverter/1 -> Concat/1
  Slice1/1 -> Concat/2
  Concat/1 -> Reinterpret/1
  Reinterpret/1 -> Out1/1

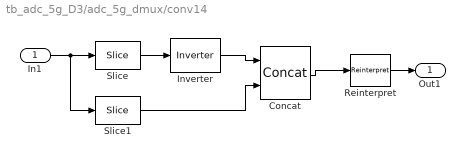
== system tb_adc_5g_D3/adc_5g_dmux/conv14 ==
  In1 : Inport  OutDataType=sfix(16)  OutScaling=2^0
  Concat : xbsIndex_r4/Concat  num_inputs=2  dbl_ovrd=off  block_type=concat
      settings: block_version=8.2.02
  Inverter : xbsIndex_r4/Inverter  en=off  latency=0  dbl_ovrd=off  block_type=inv
      settings: xl_area=[0, 0, 0, 0, 0, 0, 0]  block_version=8.2.02
  Reinterpret : xbsIndex_r4/Reinterpret  force_arith_type=on  arith_type="Signed  (2's comp)"  force_bin_pt=on  bin_pt=3  block_type=reinterpret
      settings: infoedit="Changes signal type without altering the binary representation.   You can changed the signal between signed and unsigned, and relocate the binary point.<P><P>Hardware notes: In hardware this block costs nothing.<P><P>Example:  Suppose the input is 6 bits wide, signed, with 2 fractional bits, and the output is forced to unsigned with 0 fractional bits.  Then an input of -2.0 (1110.00 in binary 2's complement) becomes an output of 56 (111000 in binary)."  block_version=8.2.02
  Slice : xbsIndex_r4/Slice  nbits=1  boolean_output=off  mode=Upper Bit Location + Width  bit1=0  base1=MSB of Input  bit0=0  base0=LSB of Input  dbl_ovrd=off  block_type=slice
      settings: infoedit="Extracts a given range of bits from each input sample and presents it at the output.  The output type is ordinarily unsigned with binary point at zero, but can be Boolean when the slice is one bit wide.<P><P>Hardware notes: In hardware this block costs nothing."  block_version=8.2.02
  Slice1 : xbsIndex_r4/Slice  nbits=3  boolean_output=off  mode=Lower Bit Location + Width  bit1=0  base1=MSB of Input  bit0=0  base0=LSB of Input  dbl_ovrd=off  block_type=slice
      settings: infoedit="Extracts a given range of bits from each input sample and presents it at the output.  The output type is ordinarily unsigned with binary point at zero, but can be Boolean when the slice is one bit wide.<P><P>Hardware notes: In hardware this block costs nothing."  block_version=8.2.02
  Out1 : Outport  OutDataType=sfix(16)  OutScaling=2^0
  wires:
  In1/1 -> Slice1/1, Slice/1
  Slice/1 -> Inverter/1
  Inverter/1 -> Concat/1
  Slice1/1 -> Concat/2
  Concat/1 -> Reinterpret/1
  Reinterpret/1 -> Out1/1

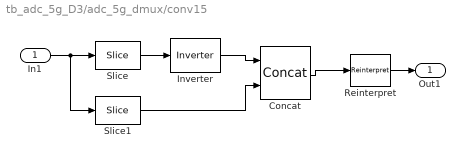
== system tb_adc_5g_D3/adc_5g_dmux/conv15 ==
  In1 : Inport  OutDataType=sfix(16)  OutScaling=2^0
  Concat : xbsIndex_r4/Concat  num_inputs=2  dbl_ovrd=off  block_type=concat
      settings: block_version=8.2.02
  Inverter : xbsIndex_r4/Inverter  en=off  latency=0  dbl_ovrd=off  block_type=inv
      settings: xl_area=[0, 0, 0, 0, 0, 0, 0]  block_version=8.2.02
  Reinterpret : xbsIndex_r4/Reinterpret  force_arith_type=on  arith_type="Signed  (2's comp)"  force_bin_pt=on  bin_pt=3  block_type=reinterpret
      settings: infoedit="Changes signal type without altering the binary representation.   You can changed the signal between signed and unsigned, and relocate the binary point.<P><P>Hardware notes: In hardware this block costs nothing.<P><P>Example:  Suppose the input is 6 bits wide, signed, with 2 fractional bits, and the output is forced to unsigned with 0 fractional bits.  Then an input of -2.0 (1110.00 in binary 2's complement) becomes an output of 56 (111000 in binary)."  block_version=8.2.02
  Slice : xbsIndex_r4/Slice  nbits=1  boolean_output=off  mode=Upper Bit Location + Width  bit1=0  base1=MSB of Input  bit0=0  base0=LSB of Input  dbl_ovrd=off  block_type=slice
      settings: infoedit="Extracts a given range of bits from each input sample and presents it at the output.  The output type is ordinarily unsigned with binary point at zero, but can be Boolean when the slice is one bit wide.<P><P>Hardware notes: In hardware this block costs nothing."  block_version=8.2.02
  Slice1 : xbsIndex_r4/Slice  nbits=3  boolean_output=off  mode=Lower Bit Location + Width  bit1=0  base1=MSB of Input  bit0=0  base0=LSB of Input  dbl_ovrd=off  block_type=slice
      settings: infoedit="Extracts a given range of bits from each input sample and presents it at the output.  The output type is ordinarily unsigned with binary point at zero, but can be Boolean when the slice is one bit wide.<P><P>Hardware notes: In hardware this block costs nothing."  block_version=8.2.02
  Out1 : Outport  OutDataType=sfix(16)  OutScaling=2^0
  wires:
  In1/1 -> Slice1/1, Slice/1
  Slice/1 -> Inverter/1
  Inverter/1 -> Concat/1
  Slice1/1 -> Concat/2
  Concat/1 -> Reinterpret/1
  Reinterpret/1 -> Out1/1

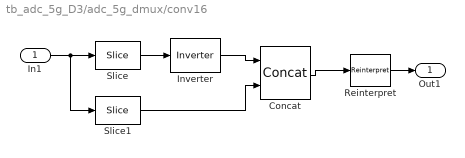
== system tb_adc_5g_D3/adc_5g_dmux/conv16 ==
  In1 : Inport  OutDataType=sfix(16)  OutScaling=2^0
  Concat : xbsIndex_r4/Concat  num_inputs=2  dbl_ovrd=off  block_type=concat
      settings: block_version=8.2.02
  Inverter : xbsIndex_r4/Inverter  en=off  latency=0  dbl_ovrd=off  block_type=inv
      settings: xl_area=[0, 0, 0, 0, 0, 0, 0]  block_version=8.2.02
  Reinterpret : xbsIndex_r4/Reinterpret  force_arith_type=on  arith_type="Signed  (2's comp)"  force_bin_pt=on  bin_pt=3  block_type=reinterpret
      settings: infoedit="Changes signal type without altering the binary representation.   You can changed the signal between signed and unsigned, and relocate the binary point.<P><P>Hardware notes: In hardware this block costs nothing.<P><P>Example:  Suppose the input is 6 bits wide, signed, with 2 fractional bits, and the output is forced to unsigned with 0 fractional bits.  Then an input of -2.0 (1110.00 in binary 2's complement) becomes an output of 56 (111000 in binary)."  block_version=8.2.02
  Slice : xbsIndex_r4/Slice  nbits=1  boolean_output=off  mode=Upper Bit Location + Width  bit1=0  base1=MSB of Input  bit0=0  base0=LSB of Input  dbl_ovrd=off  block_type=slice
      settings: infoedit="Extracts a given range of bits from each input sample and presents it at the output.  The output type is ordinarily unsigned with binary point at zero, but can be Boolean when the slice is one bit wide.<P><P>Hardware notes: In hardware this block costs nothing."  block_version=8.2.02
  Slice1 : xbsIndex_r4/Slice  nbits=3  boolean_output=off  mode=Lower Bit Location + Width  bit1=0  base1=MSB of Input  bit0=0  base0=LSB of Input  dbl_ovrd=off  block_type=slice
      settings: infoedit="Extracts a given range of bits from each input sample and presents it at the output.  The output type is ordinarily unsigned with binary point at zero, but can be Boolean when the slice is one bit wide.<P><P>Hardware notes: In hardware this block costs nothing."  block_version=8.2.02
  Out1 : Outport  OutDataType=sfix(16)  OutScaling=2^0
  wires:
  In1/1 -> Slice1/1, Slice/1
  Slice/1 -> Inverter/1
  Inverter/1 -> Concat/1
  Slice1/1 -> Concat/2
  Concat/1 -> Reinterpret/1
  Reinterpret/1 -> Out1/1

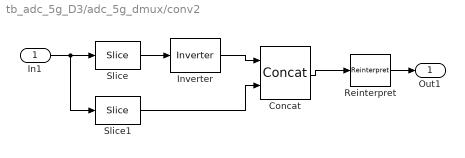
== system tb_adc_5g_D3/adc_5g_dmux/conv2 ==
  In1 : Inport  OutDataType=sfix(16)  OutScaling=2^0
  Concat : xbsIndex_r4/Concat  num_inputs=2  dbl_ovrd=off  block_type=concat
      settings: block_version=8.2.02
  Inverter : xbsIndex_r4/Inverter  en=off  latency=0  dbl_ovrd=off  block_type=inv
      settings: xl_area=[0, 0, 0, 0, 0, 0, 0]  block_version=8.2.02
  Reinterpret : xbsIndex_r4/Reinterpret  force_arith_type=on  arith_type="Signed  (2's comp)"  force_bin_pt=on  bin_pt=3  block_type=reinterpret
      settings: infoedit="Changes signal type without altering the binary representation.   You can changed the signal between signed and unsigned, and relocate the binary point.<P><P>Hardware notes: In hardware this block costs nothing.<P><P>Example:  Suppose the input is 6 bits wide, signed, with 2 fractional bits, and the output is forced to unsigned with 0 fractional bits.  Then an input of -2.0 (1110.00 in binary 2's complement) becomes an output of 56 (111000 in binary)."  block_version=8.2.02
  Slice : xbsIndex_r4/Slice  nbits=1  boolean_output=off  mode=Upper Bit Location + Width  bit1=0  base1=MSB of Input  bit0=0  base0=LSB of Input  dbl_ovrd=off  block_type=slice
      settings: infoedit="Extracts a given range of bits from each input sample and presents it at the output.  The output type is ordinarily unsigned with binary point at zero, but can be Boolean when the slice is one bit wide.<P><P>Hardware notes: In hardware this block costs nothing."  block_version=8.2.02
  Slice1 : xbsIndex_r4/Slice  nbits=3  boolean_output=off  mode=Lower Bit Location + Width  bit1=0  base1=MSB of Input  bit0=0  base0=LSB of Input  dbl_ovrd=off  block_type=slice
      settings: infoedit="Extracts a given range of bits from each input sample and presents it at the output.  The output type is ordinarily unsigned with binary point at zero, but can be Boolean when the slice is one bit wide.<P><P>Hardware notes: In hardware this block costs nothing."  block_version=8.2.02
  Out1 : Outport  OutDataType=sfix(16)  OutScaling=2^0
  wires:
  In1/1 -> Slice1/1, Slice/1
  Slice/1 -> Inverter/1
  Inverter/1 -> Concat/1
  Slice1/1 -> Concat/2
  Concat/1 -> Reinterpret/1
  Reinterpret/1 -> Out1/1

== system tb_adc_5g_D3/adc_5g_dmux/conv3 ==
  In1 : Inport  OutDataType=sfix(16)  OutScaling=2^0
  Concat : xbsIndex_r4/Concat  num_inputs=2  dbl_ovrd=off  block_type=concat
      settings: block_version=8.2.02
  Inverter : xbsIndex_r4/Inverter  en=off  latency=0  dbl_ovrd=off  block_type=inv
      settings: xl_area=[0, 0, 0, 0, 0, 0, 0]  block_version=8.2.02
  Reinterpret : xbsIndex_r4/Reinterpret  force_arith_type=on  arith_type="Signed  (2's comp)"  force_bin_pt=on  bin_pt=3  block_type=reinterpret
      settings: infoedit="Changes signal type without altering the binary representation.   You can changed the signal between signed and unsigned, and relocate the binary point.<P><P>Hardware notes: In hardware this block costs nothing.<P><P>Example:  Suppose the input is 6 bits wide, signed, with 2 fractional bits, and the output is forced to unsigned with 0 fractional bits.  Then an input of -2.0 (1110.00 in binary 2's complement) becomes an output of 56 (111000 in binary)."  block_version=8.2.02
  Slice : xbsIndex_r4/Slice  nbits=1  boolean_output=off  mode=Upper Bit Location + Width  bit1=0  base1=MSB of Input  bit0=0  base0=LSB of Input  dbl_ovrd=off  block_type=slice
      settings: infoedit="Extracts a given range of bits from each input sample and presents it at the output.  The output type is ordinarily unsigned with binary point at zero, but can be Boolean when the slice is one bit wide.<P><P>Hardware notes: In hardware this block costs nothing."  block_version=8.2.02
  Slice1 : xbsIndex_r4/Slice  nbits=3  boolean_output=off  mode=Lower Bit Location + Width  bit1=0  base1=MSB of Input  bit0=0  base0=LSB of Input  dbl_ovrd=off  block_type=slice
      settings: infoedit="Extracts a given range of bits from each input sample and presents it at the output.  The output type is ordinarily unsigned with binary point at zero, but can be Boolean when the slice is one bit wide.<P><P>Hardware notes: In hardware this block costs nothing."  block_version=8.2.02
  Out1 : Outport  OutDataType=sfix(16)  OutScaling=2^0
  wires:
  In1/1 -> Slice1/1, Slice/1
  Slice/1 -> Inverter/1
  Inverter/1 -> Concat/1
  Slice1/1 -> Concat/2
  Concat/1 -> Reinterpret/1
  Reinterpret/1 -> Out1/1
